simulink model "lab6_sec_5__PD"  (R2018a)
settings: Solver=VariableStepAuto  StartTime=0.0  StopTime=10  MaxStep=0.001  RelTol=1e-3
libraries: powerlib x4, ECEN315_Library x2, ECEN315_Library_Fault x1
settings Model: Creator=joshua  LastModifiedBy=joshua

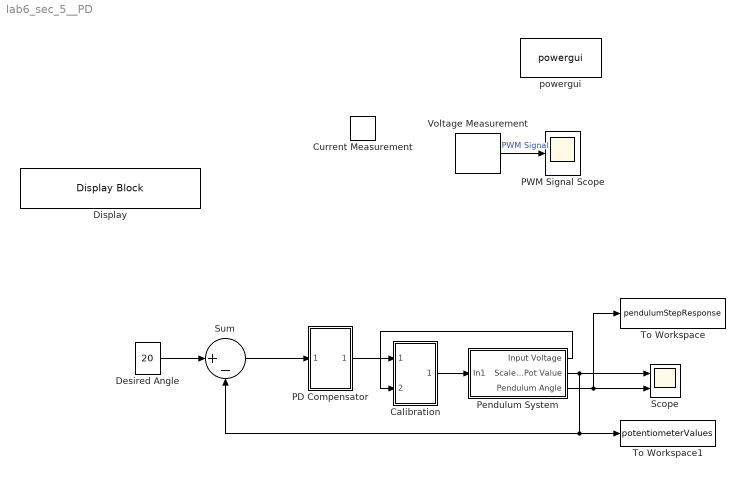
== system lab6_sec_5__PD ==
  "Calibration " : Subsystem
  Current Measurement : powerlib/Measurements/Current Measurement  PhasorSimulation=off  OutputType=Complex  PSBequivalent=0
  Desired Angle : Constant  Value=20  VectorParams1D=off  OutDataTypeStr=double
  Display : DisplayBlock  WebBlockId=38  LabelPosition=Hide
  PD Compensator : Subsystem  mask{Kp=0.1, Kd=0.13}
  PWM Signal Scope : Scope
  Pendulum System : Subsystem
  Scope : Scope  NumInputPorts=2
  Sum : Sum  Inputs=|+-
  To Workspace : ToWorkspace  VariableName=pendulumStepResponse  SampleTime=-1
      settings: Save2DSignal=2-D array (concatenate along first dimension)
  To Workspace1 : ToWorkspace  VariableName=potentiometerValues  SampleTime=-1
      settings: Save2DSignal=2-D array (concatenate along first dimension)
  Voltage Measurement : powerlib/Measurements/Voltage Measurement  PhasorSimulation=off  OutputType=Complex  PSBequivalent=0
  powergui : powerlib/powergui  Priority=1  SimulationMode=Continuous  SampleTime=50e-6  frequency=60  Iterations=50  frequencyindice=0  Pbase=100e6  ErrMax=1e-4  UnitsV=kV  UnitsW=MW  buscounter=0  FunctionMessages=off  echomessages=off  EnableUseOfTLC=off  CurrentSourceSwitches=off  DisableSnubberDevices=off  DisableRonSwitches=off  DisableVfSwitches=off  DisplayEquations=off  SolverType=Tustin/Backward Euler (TBE)  Interpol=off  ExternalGateDelay=off  methode=off  Ts=100  x0status=blocks  SPID=on  SwTol=0  HookPort=off  RestoreLinks=warning  ResistiveCurrentMeasurement=off  Frange=[0:2:500]  Ylog=off  Xlog=on  ShowGrid=off  save=off  variable=ZData  structure=0  ZoomFFT=off  StartTime=0.0  cycles=1  DisplayStyle=1  fundamental=60  FreqAxis=off  MaxFrequency=1000  frequencyindicesteady=1  RmsSteady=1  display=off
  wires:
  Voltage Measurement/1 -> PWM Signal Scope/1  "PWM Signal"
  Desired Angle/1 -> Sum/1
  Sum/1 -> PD Compensator/1(In1)
  PD Compensator/1(Out1) -> "Calibration "/1(In1)
  Pendulum System/2(Scaled Pot Value) -> Sum/2, To Workspace1/1, Scope/1
  Pendulum System/3(Pendulum Angle) -> Scope/2, To Workspace/1
  "Calibration "/1(PWM) -> Pendulum System/1(In1)
  Pendulum System/1(Input Voltage) -> "Calibration "/2(Input Voltage)

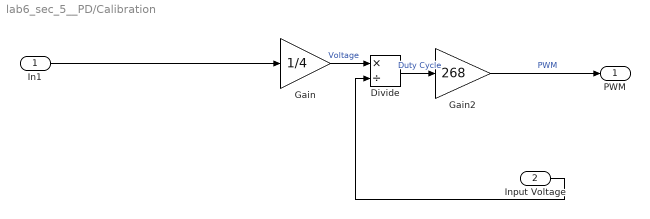
== system lab6_sec_5__PD/Calibration  ==
  In1 : Inport
  Input Voltage : Inport  Port=2
  Divide : Product  Inputs=*/
  Gain : Gain  Gain=1/4
  Gain2 : Gain  Gain=268
  PWM : Outport
  wires:
  Input Voltage/1 -> Divide/2
  Gain2/1 -> PWM/1  "PWM"
  In1/1 -> Gain/1
  Divide/1 -> Gain2/1  "Duty Cycle"
  Gain/1 -> Divide/1  "Voltage"

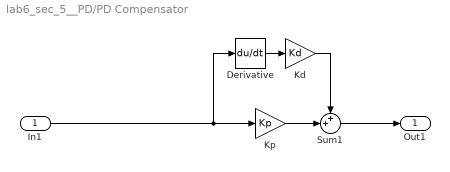
== system lab6_sec_5__PD/PD Compensator ==
  In1 : Inport
  Derivative : Derivative
  "Kd " : Gain  Gain=Kd
  "Kp " : Gain  Gain=Kp
  Sum1 : Sum  Inputs=++|
  Out1 : Outport
  wires:
  "Kp "/1 -> Sum1/2
  In1/1 -> Derivative/1, "Kp "/1
  "Kd "/1 -> Sum1/1
  Sum1/1 -> Out1/1
  Derivative/1 -> "Kd "/1

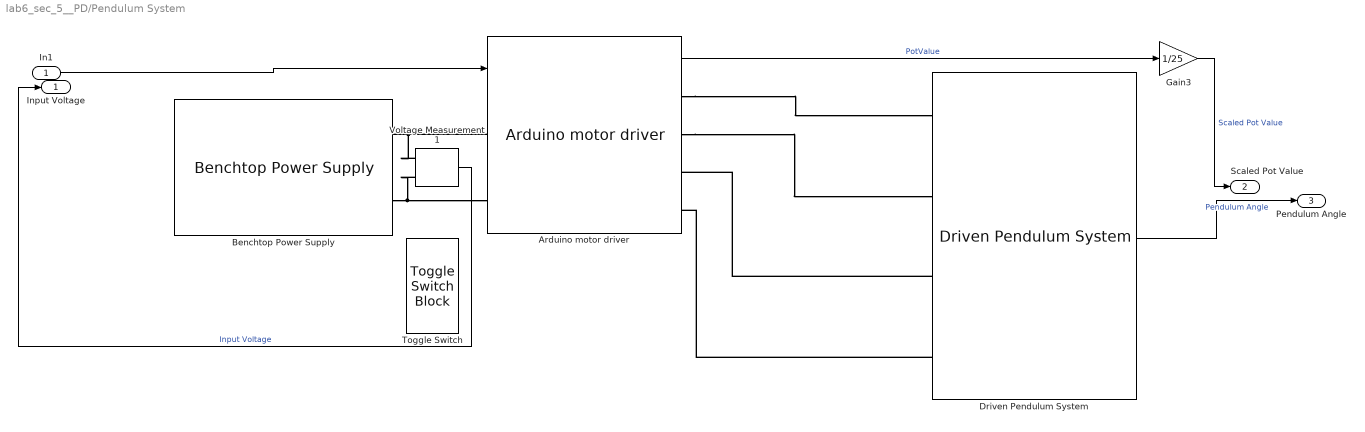
== system lab6_sec_5__PD/Pendulum System ==
  In1 : Inport
  Arduino motor driver : ECEN315_Library_Fault/Arduino motor driver  E=off
  Benchtop Power Supply : ECEN315_Library/Benchtop Power Supply  V=12
  Driven Pendulum System : ECEN315_Library/Driven Pendulum System  SystemSampleTime=-1
  Gain3 : Gain  Gain=1/25
  Toggle Switch : ToggleSwitchBlock  WebBlockId=55
      settings: Values={{'Off', 'On'}, [0 12]}
  Voltage Measurement1 : powerlib/Measurements/Voltage Measurement  PhasorSimulation=off  OutputType=Complex  PSBequivalent=0
  Input Voltage : Outport
  Scaled Pot Value : Outport  Port=2
  Pendulum Angle : Outport  Port=3
  wires:
  Arduino motor driver/1 -> Gain3/1  "PotValue"
  Gain3/1 -> Scaled Pot Value/1  "Scaled Pot Value"
  Driven Pendulum System/1 -> Pendulum Angle/1  "Pendulum Angle"
  Voltage Measurement1/1 -> Input Voltage/1  "Input Voltage"
  In1/1 -> Arduino motor driver/1
  connections:
  Driven Pendulum System/LConn3 -- Arduino motor driver/RConn3
  Arduino motor driver/RConn2 -- Driven Pendulum System/LConn2
  Benchtop Power Supply/RConn2 -- Voltage Measurement1/LConn2 -- Arduino motor driver/LConn2
  Driven Pendulum System/LConn4 -- Arduino motor driver/RConn4
  Arduino motor driver/RConn1 -- Driven Pendulum System/LConn1
  Arduino motor driver/LConn1 -- Voltage Measurement1/LConn1 -- Benchtop Power Supply/RConn1
